simulink model "discrete_event_state_mcp"  (R2020a)
settings: configuration reference "globalConfig" (kept outside this file)
InitFcn:
  | rpm=[900 1000 1100 1200 1300 1400 1500 1600 1700 1800 1900];
undefined symbols (not defined in the file): mcp_nominal_rotation, mcp_ralenti_rotation
settings Model: Creator=victo  LastModifiedBy=ToT_IPMS_03
settings ConfigSetRef: SourceName=globalConfig  SourceLocation=Base Workspace

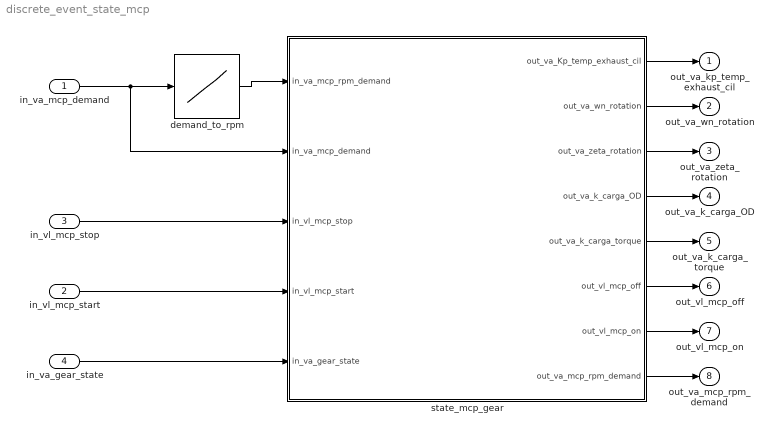
== system discrete_event_state_mcp ==
  in_va_mcp_demand : Inport  OutMin=[-100]  OutMax=[100]  OutDataTypeStr=int16  PortDimensions=1
  in_vl_mcp_start : Inport  Port=2  OutDataTypeStr=boolean
  in_vl_mcp_stop : Inport  Port=3  OutDataTypeStr=boolean
  in_va_gear_state : Inport  Port=4  OutMin=0  OutMax=2  OutDataTypeStr=uint8
  demand_to_rpm : Lookup_n-D  NumberOfTableDimensions=1  BreakpointsForDimension1=[-100,0,100]  Table=[mcp_nominal_rotation,mcp_ralenti_rotation,mcp_nominal_rotation]  ExtrapMethod=Clip  InternalRulePriority=Speed  OutDataTypeStr=uint16  RndMeth=Simplest  InputSameDT=on
  state_mcp_gear : Stateflow chart  TreatAsAtomicUnit=on
  out_va_kp_temp_exhaust_cil : Outport  OutDataTypeStr=double  PortDimensions=1  SampleTime=[0,1]
  out_va_wn_rotation : Outport  Port=2  OutDataTypeStr=double  PortDimensions=1  SampleTime=[0,1]
  out_va_zeta_rotation : Outport  Port=3  OutDataTypeStr=double  PortDimensions=1  SampleTime=[0,1]
  out_va_k_carga_OD : Outport  Port=4  OutDataTypeStr=double  PortDimensions=1  SampleTime=[0,1]
  out_va_k_carga_torque : Outport  Port=5  OutDataTypeStr=double  PortDimensions=1  SampleTime=[0,1]
  out_vl_mcp_off : Outport  Port=6  OutDataTypeStr=boolean  PortDimensions=1  SampleTime=[0,1]
  out_vl_mcp_on : Outport  Port=7  OutDataTypeStr=boolean  PortDimensions=1  SampleTime=[0,1]
  out_va_mcp_rpm_demand : Outport  Port=8  OutMin=[0]  OutMax=[mcp_nominal_rotation]  OutDataTypeStr=uint16  PortDimensions=1  SampleTime=[0,1]
  wires:
  in_va_mcp_demand/1 -> state_mcp_gear/2(in_va_mcp_demand), demand_to_rpm/1
  state_mcp_gear/1(out_va_Kp_temp_exhaust_cil) -> out_va_kp_temp_exhaust_cil/1
  state_mcp_gear/2(out_va_wn_rotation) -> out_va_wn_rotation/1
  state_mcp_gear/3(out_va_zeta_rotation) -> out_va_zeta_rotation/1
  state_mcp_gear/4(out_va_k_carga_OD) -> out_va_k_carga_OD/1
  state_mcp_gear/5(out_va_k_carga_torque) -> out_va_k_carga_torque/1
  in_vl_mcp_stop/1 -> state_mcp_gear/3(in_vl_mcp_stop)
  in_vl_mcp_start/1 -> state_mcp_gear/4(in_vl_mcp_start)
  state_mcp_gear/7(out_vl_mcp_on) -> out_vl_mcp_on/1
  state_mcp_gear/6(out_vl_mcp_off) -> out_vl_mcp_off/1
  state_mcp_gear/8(out_va_mcp_rpm_demand) -> out_va_mcp_rpm_demand/1
  demand_to_rpm/1 -> state_mcp_gear/1(in_va_mcp_rpm_demand)
  in_va_gear_state/1 -> state_mcp_gear/5(in_va_gear_state)

== stateflow chart discrete_event_state_mcp/state_mcp_gear ==
  state mcp_status [parallel]
    settings: executionOrder=1
    state off
      entry:
      out_vl_mcp_on=false;
      out_vl_mcp_off=true;
      out_va_mcp_rpm_demand =0;
    state on
      entry , during:
      out_vl_mcp_on = true;
      out_vl_mcp_off = false;
      out_va_mcp_rpm_demand = in_va_mcp_rpm_demand;
    (default) -> off
    off -> on : [in_vl_mcp_start==1]
    on -> off : [in_vl_mcp_stop==1]
  state gear_position [parallel]
    settings: executionOrder=2
    state astern
      entry:
      out_va_Kp_temp_exhaust_cil=69.8/200;
      out_va_wn_rotation=0.5;
      out_va_zeta_rotation=0.9;
      out_va_k_carga_OD=1.2;
      out_va_k_carga_torque=1;
    state ahead
      entry:
      out_va_Kp_temp_exhaust_cil=69.8/200;
      out_va_wn_rotation=1.2;
      out_va_zeta_rotation=0.9;
      out_va_k_carga_OD=1.2;
      out_va_k_carga_torque=1;
    state neutral
      entry:
      out_va_Kp_temp_exhaust_cil=10/1300;
      out_va_wn_rotation=1.2;
      out_va_zeta_rotation=0.7;
      out_va_k_carga_OD=1;
      out_va_k_carga_torque=0.67;
    (default) -> neutral
    neutral -> astern [order 2] : [in_va_mcp_demand<0&& in_va_gear_state==2]
    neutral -> ahead [order 1] : [in_va_mcp_demand>0 && in_va_gear_state==1]
    astern -> neutral : [in_va_gear_state~=2]
    ahead -> neutral : [in_va_gear_state~=1]
  note: TODO:
      | 1. Inserir a interface do sinal do estado da ER.
      | 2. Avaliar se é melhor utilizar um bool para o estado da ER.
  data: out_va_Kp_temp_exhaust_cil output double; out_va_wn_rotation output double; out_va_zeta_rotation output double; out_va_k_carga_OD output double; out_va_k_carga_torque output; out_vl_mcp_off output boolean; in_va_mcp_rpm_demand input uint16; in_va_mcp_demand input int16; in_vl_mcp_stop input boolean; in_vl_mcp_start input boolean; out_vl_mcp_on output boolean; out_va_mcp_rpm_demand output uint16; in_va_gear_state input uint8
